simulink model "DD_4W_model"  (R2020b)
settings: Solver=VariableStepAuto  StartTime=0.0  StopTime=5  RelTol=1e-3
values from neighbouring files (symbols this model uses):
  a = 0.37    [main.m]
  b = 0.55    [main.m]
  fr_act = 0.12    [main.m]
  g = 9.81    [main.m]
  M = [m 0 0; 0 m 0; 0 0 I]    [main.m]
  m = 116    [main.m]
  mu_act = 0.88    [main.m]
  q0 = [0;0;deg2rad(10)]    [main.m]
  q0_dot = [[cos(q0(3)) -sin(q0(3));sin(q0(3)) cos(q0(3))]*[0.5;0.5];-2.2]    [main.m]
  r = 0.2    [main.m]
settings Model: Creator=sumit  LastModifiedBy=sumit

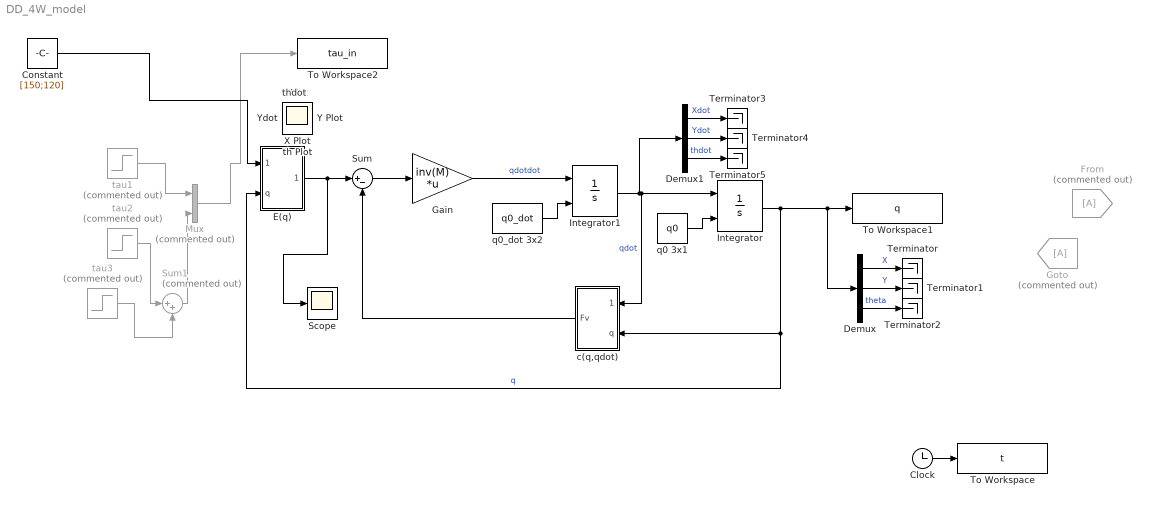
== system DD_4W_model ==
  Clock : Clock
  Constant : Constant  Value=[150;120]
  Demux : Demux  Outputs=3
  Demux1 : Demux  Outputs=3
  E(q) : Subsystem
  From : From  Commented=on
  Gain : Gain  Gain=inv(M)  Multiplication=Matrix(K*u)
  Goto : Goto  Commented=on
  Integrator : Integrator  InitialConditionSource=external
  Integrator1 : Integrator  InitialConditionSource=external
  Mux : Mux  Commented=on  Inputs=2
  Scope : Scope
  Sum : Sum  Inputs=|+-
  Sum1 : Sum  Commented=on  Inputs=|++
  Terminator{,1..5} (6 alike) : Terminator
  To Workspace : ToWorkspace  VariableName=t  SampleTime=-1
  To Workspace1 : ToWorkspace  VariableName=q  SampleTime=-1
  To Workspace2 : ToWorkspace  VariableName=tau_in  SaveFormat=Timeseries  SampleTime=-1
  c(q,qdot) : Subsystem
  q0 3x1 : Constant  Value=q0
  q0_dot 3x2 : Constant  Value=q0_dot
  tau1 : Step  Commented=on  After=120  SampleTime=0
  tau2 : Step  Commented=on  After=120  SampleTime=0
  tau3 : Step  Commented=on  Time=2  After=60  SampleTime=0
  X Plot : Scope
  Xdot : Scope
  Y Plot : Scope
  Ydot : Scope
  th Plot : Scope
  thdot : Scope
  wires:
  q0 3x1/1 -> Integrator/2
  q0_dot 3x2/1 -> Integrator1/2
  Gain/1 -> Integrator1/1  "qdotdot"
  Clock/1 -> To Workspace/1
  Integrator/1 -> c(q,qdot)/2(q), E(q)/2(q), Demux/1, To Workspace1/1  "q"
  Sum/1 -> Gain/1
  c(q,qdot)/1(Fv) -> Sum/2
  tau1/1 -> Mux/1
  tau2/1 -> Sum1/1
  Mux/1 -> To Workspace2/1
  E(q)/1(Ftau) -> Scope/1, Sum/1
  Demux/1 -> Terminator/1  "X"
  Demux/2 -> Terminator1/1  "Y"
  Demux/3 -> Terminator2/1  "theta"
  Demux1/2 -> Terminator4/1  "Ydot"
  Integrator1/1 -> Demux1/1, c(q,qdot)/1(qdot), Integrator/1  "qdot"
  Demux1/3 -> Terminator5/1  "thdot"
  Demux1/1 -> Terminator3/1  "Xdot"
  tau3/1 -> Sum1/2
  Sum1/1 -> Mux/2
  Constant/1 -> E(q)/1(tau)

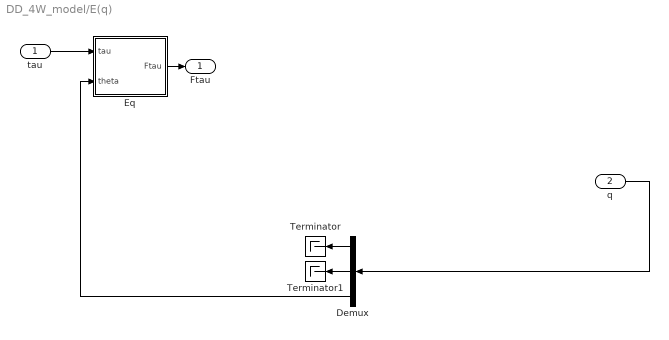
== system DD_4W_model/E(q) ==
  tau : Inport
  q : Inport  Port=2
  Demux : Demux  Outputs=3
  Eq : MATLAB Function  TreatAsAtomicUnit=on
  Terminator : Terminator
  Terminator1 : Terminator
  Ftau : Outport
  wires:
  Demux/1 -> Terminator/1
  Eq/1(Ftau) -> Ftau/1
  q/1 -> Demux/1
  Demux/2 -> Terminator1/1
  tau/1 -> Eq/1(tau)
  Demux/3 -> Eq/2(theta)

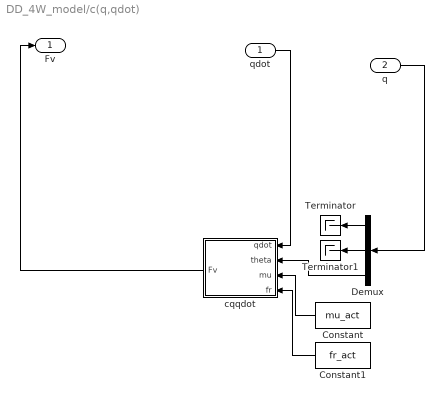
== system DD_4W_model/c(q,qdot) ==
  qdot : Inport
  q : Inport  Port=2
  Constant : Constant  Value=mu_act
  Constant1 : Constant  Value=fr_act
  Demux : Demux  Outputs=3
  Terminator : Terminator
  Terminator1 : Terminator
  cqqdot : MATLAB Function  TreatAsAtomicUnit=on
  Fv : Outport
  wires:
  Demux/2 -> Terminator1/1
  cqqdot/1(Fv) -> Fv/1
  qdot/1 -> cqqdot/1(qdot)
  Constant1/1 -> cqqdot/4(fr)
  Demux/1 -> Terminator/1
  Constant/1 -> cqqdot/3(mu)
  Demux/3 -> cqqdot/2(theta)
  q/1 -> Demux/1

== matlab function DD_4W_model/E(q)/Eq ==
  data: tau input; theta input; Ftau output; t parameter; r parameter
function Ftau = Eq(tau,theta,t, r)
Ftau=[cos(theta)/r cos(theta)/r;...
   sin(theta)/r sin(theta)/r;...
   t/r -t/r]*tau;

== matlab function DD_4W_model/c(q,qdot)/cqqdot ==
  data: qdot input; theta input; Fv output; mu input; fr input; a parameter; b parameter; t parameter; g parameter; m parameter
function Fv = cqqdot(qdot,theta,mu,fr,a, b, t, g, m)
Xdot=qdot(1);
Ydot=qdot(2);
thdot=qdot(3);

%Rth = [cos(theta) -sin(theta);sin(theta) cos(theta)];

xdot =  Xdot*cos(theta)+Ydot*sin(theta);
ydot = -Xdot*sin(theta)+Ydot*cos(theta);

x1dot = xdot-t*thdot;
x2dot = xdot+t*thdot;
y1dot = ydot-a*thdot;
y3dot = ydot+b*thdot;

Rx = fr*m*g*0.5*(sign(x1dot)+sign(x2dot));
Fy = mu*m*g*(b*sign(y1dot)+a*sign(y3dot))/(a+b);
Mr = mu*a*b*m*g*(sign(y1dot)-sign(y3dot))/(a+b)...
     + fr*t*m*g*0.5*(sign(x2dot)-sign(x1dot));
 
Fv=[Rx*cos(theta)-Fy*sin(theta);...
   Rx*sin(theta)+Fy*cos(theta);...
   Mr];
